simulink model "sample01_current_I2C1"  (R2025a)
settings: Solver=ode1  StartTime=0.0  StopTime=inf  FixedStep=0.005  RelTol=1e-3  EnableMultiTasking=on
libraries: roller485lib x3
settings Model: SILPILModeSetting=veronly  ExtModeTrigDuration=2  Creator=kawata  LastModifiedBy=kawata
settings SolverCC: AutoInsertRateTranBlk=on
settings DataIOCC: ReturnWorkspaceOutputs=off
settings OptimizationCC: EnhancedBackFolding=on  PassReuseOutputArgsThreshold=0.0  MaxStackSize=64  OptimizeBlockOrder=speed  DifferentSizesBufferReuse=on  OptimizationCustomize=off
settings DebuggingCC: ParameterTunabilityLossMsg=error
settings HardwareCC: ProdBitPerPointer=32.0  ProdBitPerSizeT=32.0  ProdBitPerPtrDiffT=32.0  ProdLargestAtomicInteger=Long  ProdLargestAtomicFloat=Double  ProdWordSize=32.0  ProdHWDeviceType=ARM Compatible->ARM Cortex  UseEmbeddedCoderFeatures=off  UseSimulinkCoderFeatures=off
settings SFSimCC: MATLABDynamicMemAlloc=off
settings RTWCC: SystemTargetFile=ert.tlc  HardwareBoard=Raspberry Pi Pico (Arduino Compatible)  TemplateMakefile=ert_default_tmf  Toolchain=Arduino ARM RP2040  BuildConfiguration=Faster Runs  Description=Embedded Coder
settings CodeAppCC: ForceParamTrailComments=on  OperatorAnnotations=on
settings ERTTargetCC: ExtModeTransport=3.0  ExtModeAutomaticAllocSize=off  ExtModeStaticAllocSize=65536.0  InlinedParameterPlacement=Hierarchical  DynamicArrayContainerType=coder::array  ERTCustomFileBanners=off  SupportContinuousTime=on  SupportNonInlinedSFcns=on  RemoveResetFunc=off  SupportVariableSizeSignals=on  ModelStepFunctionPrototypeControlCompliant=off

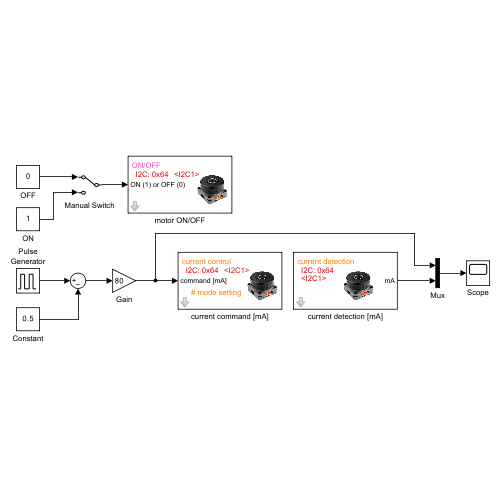
[thumbnail: Simulink's stored preview of the top-level diagram]
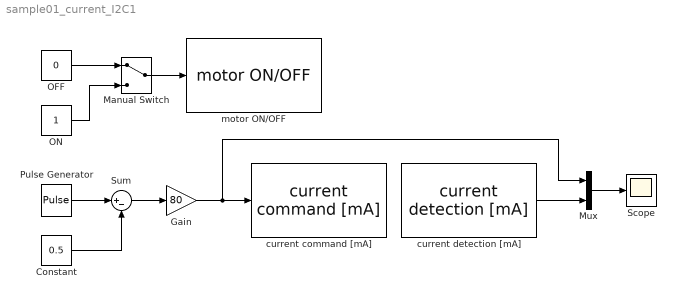
== system sample01_current_I2C1 ==
  Constant : Constant  Value=0.5
  Gain : Gain  Gain=80
  Manual Switch : ManualSwitch
  Mux : Mux  Inputs=2
  OFF : Constant  Value=0
  ON : Constant
  Pulse Generator : DiscretePulseGenerator  PulseType=Time based  Period=4  PulseWidth=50  PhaseDelay=1
  Scope : Scope
      settings: TimeSpan=4  ActiveDisplayYMinimum=-80  ActiveDisplayYMaximum=80
  Sum : Sum  Inputs=|+-
  current command [mA] : roller485lib/I2C Write/current command [mA]  I2CAddress=0x64  I2CModule=1  set_time=0
      settings: SourceProductName=Roller485 Library
  current detection [mA] : roller485lib/I2C Read/current detection [mA]  I2CAddress=0x64  I2CModule=1  sample_time=-1
      settings: SourceProductName=Roller485 Library
  motor ON/OFF : roller485lib/motor ON//OFF  I2CAddress=0x64  I2CModule=1
      settings: SourceProductName=Roller485 Library
  wires:
  Manual Switch/1 -> motor ON/OFF/1
  OFF/1 -> Manual Switch/1
  ON/1 -> Manual Switch/2
  Gain/1 -> current command [mA]/1, Mux/1
  Sum/1 -> Gain/1
  Constant/1 -> Sum/2
  Pulse Generator/1 -> Sum/1
  current detection [mA]/1 -> Mux/2
  Mux/1 -> Scope/1
